simulink model "SYS"  (R2015a)
settings: Solver=ode45  StartTime=0.0  StopTime=T  RelTol=1e-3
values from neighbouring files (symbols this model uses):
  fs = 100    [validation.m]
undefined symbols (not defined in the file or in its folder): Atrue, Btrue, Ctrue, Dtrue
settings Model: Creator=Diogo  LastModifiedBy=Diogo

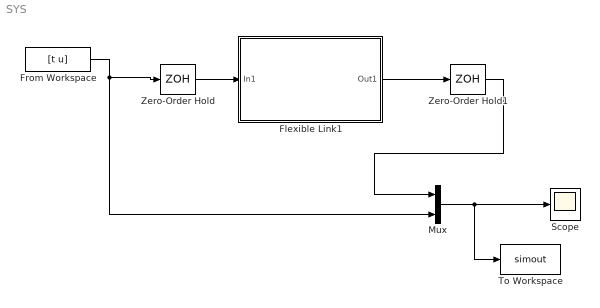
== system SYS ==
  Flexible Link1 : Subsystem
      mask Display: image('quanserlink.jpg')
  From Workspace : FromWorkspace  VariableName=[t u]  SampleTime=0
  Mux : Mux  Inputs=2
  Scope : Scope
  To Workspace : ToWorkspace  VariableName=simout  SaveFormat=Structure With Time  SampleTime=-1
  Zero-Order Hold : ZeroOrderHold  SampleTime=1/fs
  Zero-Order Hold1 : ZeroOrderHold  SampleTime=1/fs
  wires:
  From Workspace/1 -> Mux/2, Zero-Order Hold/1
  Mux/1 -> To Workspace/1, Scope/1
  Zero-Order Hold/1 -> Flexible Link1/1(In1)
  Flexible Link1/1(Out1) -> Zero-Order Hold1/1
  Zero-Order Hold1/1 -> Mux/1

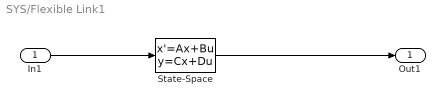
== system SYS/Flexible Link1 ==
  In1 : Inport
  State-Space : StateSpace  A=Atrue  B=Btrue  C=Ctrue  D=Dtrue  X0=0
  Out1 : Outport
  wires:
  State-Space/1 -> Out1/1
  In1/1 -> State-Space/1
